simulink model "mfordmodel_v1"  (R2023a)
settings: Solver=ode45  StartTime=0.0  StopTime=10.0  RelTol=1e-3  EnableMultiTasking=on
undefined symbols (not defined in the file): ABV_RATIO_SW, AC_OFF_DLY, ACLOD, AUTO_TRNS_SW, BRAKE_DNDT_X, BZZRPM, BZZRPM_ALT, BZZTM, BZZTM_ALT, CMD_LITOFF, CMD_STABLE, CO_ST_ECT__A, COOL_BASE, DAS_BKDLY_A, DAS_CNT, DAS_CTDLY, DAS_LC_SW__A, DASCLP_5INH, DASCTL, DASMHYST, DASMPH, DEBYCP, DES_BASE, DPNEU_MUL, DSDRPM_DN_TC, DSDRPM_OFF, DSDRPM_UP_TC, EDF_DELAY, EDFHP, ETC_CL_TP, ETC_HP, GR_CM_CREEP, HCAM_ACT_CLP, HEDFHP, HEDFRPM, HICAM_PS, IAC_CAL_SW, IAC_ER_TM1, IAC_ER_TM2, IAC_ER_TM4, IAC_HI_LIM__A, IAC_ISFL_OBD, IAC_KAM_SW, IAC_LO_LIM__A, IAC_MON_TM, IAC_OT_REQ, IAC_RUN_TM, IAC_TP_OBD, IAC_TR_DAS, IAC_TST_DC, ID_DAS__A, ID_NOVS__A, IDVS_CH__A, IDVS_SL__A, IPSI_SW, IPSIDLY, IS_DRBASE__A, IS_DRBASE_A__A, IS_NUBASE__A, IS_NUBASE_A__A ... (+35)
libraries: simulink x2
(part 7 of 12)

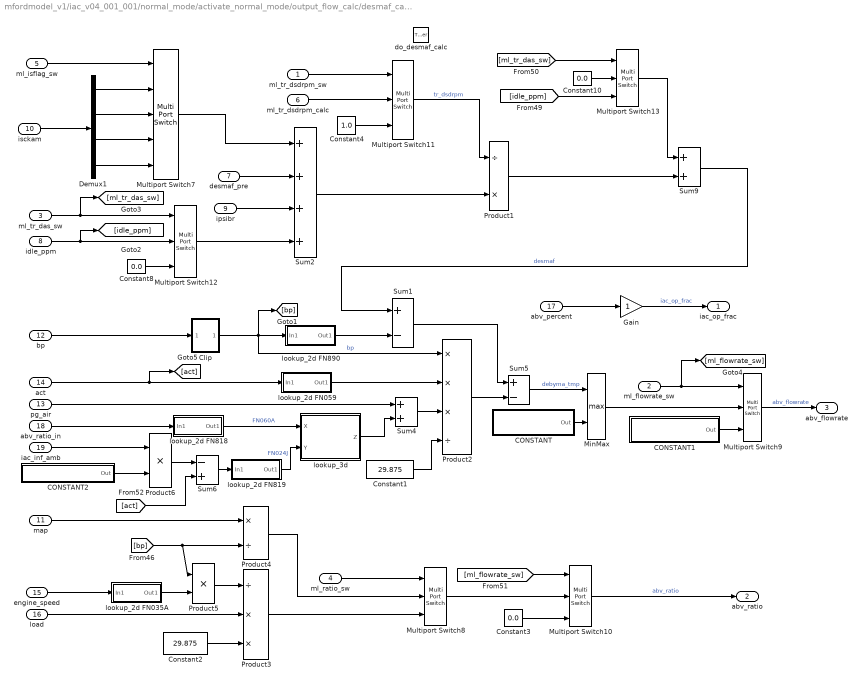
== system mfordmodel_v1/iac_v04_001_001/normal_mode/activate_normal_mode/output_flow_calc/desmaf_calc ==
  ml_tr_dsdrpm_sw : Inport
  ml_flowrate_sw : Inport  Port=2
  ml_tr_das_sw : Inport  Port=3
  ml_ratio_sw : Inport  Port=4
  ml_isflag_sw : Inport  Port=5
  ml_tr_dsdrpm_calc : Inport  Port=6
  desmaf_pre : Inport  Port=7
  idle_ppm : Inport  Port=8
  ipsibr : Inport  Port=9
  isckam : Inport  Port=10
  map : Inport  Port=11
  bp : Inport  Port=12
  pg_air : Inport  Port=13
  act : Inport  Port=14
  engine_speed : Inport  Port=15
  load : Inport  Port=16
  abv_percent : Inport  Port=17
  abv_ratio_in : Inport  Port=18
  iac_inf_amb : Inport  Port=19
  do_desmaf_calc : TriggerPort  TriggerType=function-call  VariantControl=(inherit)
  CONSTANT : Subsystem  mask(Constant){constant=DEBYCP}
      mask help: Constant Block. Will dispaly constant name and value on the icon of the block
      mask init:
      | if isletter(constant(1))
      |   const = evalin('base',constant);
      |   name = constant;
      | else
      |   const = str2num(constant);
      |   name = 'CONST';
      | end;
      mask Display: fprintf('%s = %.4f',name,const);
  CONSTANT1 : Subsystem  mask(Constant){constant=IAC_FM_PPM}
      mask help: Constant Block. Will dispaly constant name and value on the icon of the block
      mask init:
      | if isletter(constant(1))
      |   const = evalin('base',constant);
      |   name = constant;
      | else
      |   const = str2num(constant);
      |   name = 'CONST';
      | end;
      mask Display: fprintf('%s = %.4f',name,const);
  CONSTANT2 : Subsystem  mask(Constant){constant=LK_AMB_FRAC}
      mask help: Constant Block. Will dispaly constant name and value on the icon of the block
      mask init:
      | if isletter(constant(1))
      |   const = evalin('base',constant);
      |   name = constant;
      | else
      |   const = str2num(constant);
      |   name = 'CONST';
      | end;
      mask Display: fprintf('%s = %.4f',name,const);
  Clip : Subsystem  mask(Clip){max=40, min=.1, labels=on}
      mask prompts: max "Upper Limit"; min "Lower Limit"; labels "Show clip values"
      mask help:
      | Limits input signal to the upper and lower saturation
      | values.
      mask init:
      | if (labels == 1)
      |   up_label = num2str(max, '%5.3g');
      |   low_label = num2str(min, '%5.3g');
      | else
      |   up_label = ' ';
      |   low_label = ' ';
      | end
      mask Help:
      | Upper limit  -  The upper bound on the input signal.  While the signal is above this value, the block output is set to this value.
      | 
      | Lower limit  -  The lower bound on the input signal.  While the signal is below this value, the block output is set to this value.
      | 
      | Show clip values  -  If the box is checked, clip values are displayed in the icon box.
      mask Display:
      | plot( [0.1 0.3 0.7 0.9], [0.2 0.2 0.8 0.8])
      | text(0.2, 0.05, low_label)
      | text(0.7, 0.95, up_label)
  Constant1 : Constant  Value=29.875
  Constant10 : Constant  Value=0.0
  Constant2 : Constant  Value=29.875
  Constant3 : Constant  Value=0.0
  Constant4 : Constant  Value=1.0
  Constant8 : Constant  Value=0.0
  Demux1 : Demux
      settings: DisplayOption=none
  Gain : Gain  SaturateOnIntegerOverflow=on  OutDataTypeStr=Inherit: Same as input  ParamDataTypeStr=Inherit: Same as input
  MinMax : MinMax  Function=max  Inputs=2  InputSameDT=on  SaturateOnIntegerOverflow=on
  Multiport Switch{8..13} (6 alike) : MultiPortSwitch  Inputs=2
  Multiport Switch7 : MultiPortSwitch  Inputs=4
  Product1 : Product  Inputs=/*  InputSameDT=on  RndMeth=Zero  SaturateOnIntegerOverflow=on  OutDataTypeStr=Inherit: Same as first input
  Product2 : Product  Inputs=***/  InputSameDT=on  RndMeth=Zero  SaturateOnIntegerOverflow=on  OutDataTypeStr=Inherit: Same as first input
  Product3 : Product  Inputs=/**  InputSameDT=on  RndMeth=Zero  SaturateOnIntegerOverflow=on  OutDataTypeStr=Inherit: Same as first input
  Product4 : Product  Inputs=*/  InputSameDT=on  RndMeth=Zero  SaturateOnIntegerOverflow=on  OutDataTypeStr=Inherit: Same as first input
  Product5 : Product  Inputs=**  InputSameDT=on  RndMeth=Zero  SaturateOnIntegerOverflow=on  OutDataTypeStr=Inherit: Same as first input
  Product6 : Product  Inputs=**  InputSameDT=on  RndMeth=Zero  SaturateOnIntegerOverflow=on  OutDataTypeStr=Inherit: Same as first input
  Sum1 : Sum  Inputs=+-  InputSameDT=on  SaturateOnIntegerOverflow=on  OutDataTypeStr=Inherit: Same as first input
  Sum2 : Sum  Inputs=++++  InputSameDT=on  SaturateOnIntegerOverflow=on  OutDataTypeStr=Inherit: Same as first input
  Sum4 : Sum  InputSameDT=on  SaturateOnIntegerOverflow=on  OutDataTypeStr=Inherit: Same as first input
  Sum5 : Sum  Inputs=+-  InputSameDT=on  SaturateOnIntegerOverflow=on  OutDataTypeStr=Inherit: Same as first input
  Sum6 : Sum  Inputs=-+  InputSameDT=on  SaturateOnIntegerOverflow=on  OutDataTypeStr=Inherit: Same as first input
  Sum9 : Sum  InputSameDT=on  SaturateOnIntegerOverflow=on  OutDataTypeStr=Inherit: Same as first input
  lookup_2d FN035A : Subsystem  mask(2-D, piece-wise, linear interpolation){CAL_FUNC=FN035A}
      mask prompts: CAL_FUNC "Calibration function name"
      mask help:
      | Performs piece-wise linear interpolation.
      |
      | Output is NOT extrapolated beyond the input range.  If the input value presented to the block lies outside the range specified in the block's parameter, then the value is treated as though it has the value of the nearest value in the range.
      mask init: same as mfordmodel_v1/iac_v04_001_001/activate_desired_rpm/rpm_calcs/lookup_2d
      mask Help:
      | Enter the name of the calibration function.
      | (e.g. EGM_VA_ECT_MULT)
      mask Display:
      | fprintf('%s',CAL_FUNC);
      | plot(calfunc.X,calfunc.Y,max_x*1.05,max_y*1.05,min_x,min_y);
  lookup_2d FN059 : Subsystem  mask(2-D, piece-wise, linear interpolation){CAL_FUNC=FN059}
      mask prompts: CAL_FUNC "Calibration function name"
      mask help:
      | Performs piece-wise linear interpolation.
      |
      | Output is NOT extrapolated beyond the input range.  If the input value presented to the block lies outside the range specified in the block's parameter, then the value is treated as though it has the value of the nearest value in the range.
      mask init: same as mfordmodel_v1/iac_v04_001_001/activate_desired_rpm/rpm_calcs/lookup_2d
      mask Help:
      | Enter the name of the calibration function.
      | (e.g. EGM_VA_ECT_MULT)
      mask Display:
      | fprintf('%s',CAL_FUNC);
      | plot(calfunc.X,calfunc.Y,max_x*1.05,max_y*1.05,min_x,min_y);
  lookup_2d FN818 : Subsystem  mask(2-D, piece-wise, linear interpolation){CAL_FUNC=FN060A}
      mask prompts: CAL_FUNC "Calibration function name"
      mask help:
      | Performs piece-wise linear interpolation.
      |
      | Output is NOT extrapolated beyond the input range.  If the input value presented to the block lies outside the range specified in the block's parameter, then the value is treated as though it has the value of the nearest value in the range.
      mask init: same as mfordmodel_v1/iac_v04_001_001/activate_desired_rpm/rpm_calcs/lookup_2d
      mask Help:
      | Enter the name of the calibration function.
      | (e.g. EGM_VA_ECT_MULT)
      mask Display:
      | fprintf('%s',CAL_FUNC);
      | plot(calfunc.X,calfunc.Y,max_x*1.05,max_y*1.05,min_x,min_y);
  lookup_2d FN819 : Subsystem  mask(2-D, piece-wise, linear interpolation){CAL_FUNC=FN024J}
      mask prompts: CAL_FUNC "Calibration function name"
      mask help:
      | Performs piece-wise linear interpolation.
      |
      | Output is NOT extrapolated beyond the input range.  If the input value presented to the block lies outside the range specified in the block's parameter, then the value is treated as though it has the value of the nearest value in the range.
      mask init: same as mfordmodel_v1/iac_v04_001_001/activate_desired_rpm/rpm_calcs/lookup_2d
      mask Help:
      | Enter the name of the calibration function.
      | (e.g. EGM_VA_ECT_MULT)
      mask Display:
      | fprintf('%s',CAL_FUNC);
      | plot(calfunc.X,calfunc.Y,max_x*1.05,max_y*1.05,min_x,min_y);
  lookup_2d FN890 : Subsystem  mask(2-D, piece-wise, linear interpolation){CAL_FUNC=FN890}
      mask prompts: CAL_FUNC "Calibration function name"
      mask help:
      | Performs piece-wise linear interpolation.
      |
      | Output is NOT extrapolated beyond the input range.  If the input value presented to the block lies outside the range specified in the block's parameter, then the value is treated as though it has the value of the nearest value in the range.
      mask init: same as mfordmodel_v1/iac_v04_001_001/activate_desired_rpm/rpm_calcs/lookup_2d
      mask Help:
      | Enter the name of the calibration function.
      | (e.g. EGM_VA_ECT_MULT)
      mask Display:
      | fprintf('%s',CAL_FUNC);
      | plot(calfunc.X,calfunc.Y,max_x*1.05,max_y*1.05,min_x,min_y);
  lookup_3d : Subsystem  mask(3-D, piece-wise, linear interpolation){CAL_TABLE=FN8180}
      mask prompts: CAL_TABLE "Calibration table name"
      mask help:
      | Performs 3-D, piece-wise linear interpolation.
      |
      | Output is NOT extrapolated beyond the input ranges.  If an input value presented to the block lies outside the range specified in the block's parameters, then the value is treated as though it has the value of the nearest value in the range.
      mask init: same as mfordmodel_v1/iac_v04_001_001/normal_mode/activate_feedforward/desmaf_pre_calc/FN1862AD
      mask Help: Enter the name of the calibration table.
      mask Display:
      | fprintf('%s',CAL_TABLE);
      | plot(caltable.Z');
      | plot([min_x max_x],[minz*.99 minz*.99]);
      | plot([min_x min_x],[minz*.99 maxz*1.01]);
  iac_op_frac : Outport
  abv_ratio : Outport  Port=2
  abv_flowrate : Outport  Port=3
  wires:
  Multiport Switch7/1 -> Sum2/1
  Demux1/1 -> Multiport Switch7/2
  Demux1/2 -> Multiport Switch7/3
  Demux1/3 -> Multiport Switch7/4
  Demux1/4 -> Multiport Switch7/5
  ml_isflag_sw/1 -> Multiport Switch7/1
  isckam/1 -> Demux1/1
  Constant8/1 -> Multiport Switch12/3
  desmaf_pre/1 -> Sum2/2
  Multiport Switch11/1 -> Product1/1  "tr_dsdrpm"
  Sum2/1 -> Product1/2
  ipsibr/1 -> Sum2/3
  Multiport Switch13/1 -> Sum9/1
  Product1/1 -> Sum9/2
  Multiport Switch12/1 -> Sum2/4
  Constant10/1 -> Multiport Switch13/2
  [idle_ppm] -> Multiport Switch13/3
  Constant4/1 -> Multiport Switch11/3
  ml_tr_dsdrpm_sw/1 -> Multiport Switch11/1
  ml_tr_dsdrpm_calc/1 -> Multiport Switch11/2
  [ml_tr_das_sw] -> Multiport Switch13/1
  ml_tr_das_sw/1 -> Multiport Switch12/1, [ml_tr_das_sw]
  idle_ppm/1 -> [idle_ppm], Multiport Switch12/2
  ml_ratio_sw/1 -> Multiport Switch8/1
  Product4/1 -> Multiport Switch8/2
  Product3/1 -> Multiport Switch8/3
  Multiport Switch8/1 -> Multiport Switch10/2
  [ml_flowrate_sw] -> Multiport Switch10/1
  Constant3/1 -> Multiport Switch10/3
  map/1 -> Product4/1
  Product5/1 -> Product3/1
  [bp] -> Product4/2, Product5/1
  load/1 -> Product3/2
  engine_speed/1 -> lookup_2d FN035A/1(In1)
  Constant2/1 -> Product3/3
  lookup_2d FN035A/1(Out1) -> Product5/2
  Multiport Switch10/1 -> abv_ratio/1  "abv_ratio"
  MinMax/1 -> Multiport Switch9/2
  CONSTANT1/1(Out) -> Multiport Switch9/3
  Multiport Switch9/1 -> abv_flowrate/1  "abv_flowrate"
  Sum5/1 -> MinMax/1  "debyma_tmp"
  CONSTANT/1(Out) -> MinMax/2
  Product2/1 -> Sum5/2
  Sum1/1 -> Sum5/1
  lookup_2d FN890/1(Out1) -> Sum1/2
  Constant1/1 -> Product2/4
  Sum9/1 -> Sum1/1  "desmaf"
  ml_flowrate_sw/1 -> Multiport Switch9/1, [ml_flowrate_sw]
  Sum4/1 -> Product2/3
  pg_air/1 -> Sum4/1
  lookup_2d FN059/1(Out1) -> Product2/2
  bp/1 -> Clip/1(In1)
  Clip/1(Out1) -> [bp], Product2/1, lookup_2d FN890/1(In1)  "bp"
  abv_ratio_in/1 -> lookup_2d FN818/1(In1)
  lookup_3d/1(Z) -> Sum4/2
  lookup_2d FN818/1(Out1) -> lookup_3d/1(X)  "FN060A"
  act/1 -> lookup_2d FN059/1(In1), [act]
  iac_inf_amb/1 -> Product6/1
  Product6/1 -> Sum6/1
  [act] -> Sum6/2
  Sum6/1 -> lookup_2d FN819/1(In1)
  lookup_2d FN819/1(Out1) -> lookup_3d/2(Y)  "FN024J"
  Gain/1 -> iac_op_frac/1  "iac_op_frac"
  abv_percent/1 -> Gain/1
  CONSTANT2/1(Out) -> Product6/2

== system mfordmodel_v1/iac_v04_001_001/normal_mode/activate_normal_mode/output_flow_calc/tr_dsdrpm_calc ==
  tr_abs : Inport
  tr_res : Inport  Port=2
  do_tr_dsdrpm_calc : TriggerPort  TriggerType=function-call  VariantControl=(inherit)
  Sum1 : Sum  Inputs=+-  InputSameDT=on  SaturateOnIntegerOverflow=on  OutDataTypeStr=Inherit: Same as first input
  ml_tr_dsdrpm_calc : Outport  InitialOutput=0
  wires:
  tr_abs/1 -> Sum1/1
  Sum1/1 -> ml_tr_dsdrpm_calc/1  "ml_tr_dsdrpm_calc"
  tr_res/1 -> Sum1/2

== system mfordmodel_v1/iac_v04_001_001/normal_mode/iscflg_module/das_min_clip/functions ==
  n_ratch : Inport
  dasl_min_clp : Inport  Port=2
  iac_dlt_time : Inport  Port=3
  dsdrpm : Inport  Port=4
  do_functions : TriggerPort  TriggerType=function-call  VariantControl=(inherit)
  ROLAV_TC_DT_in1 : Subsystem  mask(Rolling Average - Time Constant){TAU=TC_DAS_CLPUC}
      mask prompts: TAU "Time Constant"
      mask help: Rolling Average - Time Constant. This filter block is the first order approximation using a time constant. Inputs include the time constant (entered through this dialogue), old_ave which is the previous average value, new_value which is the new filter to filter toward, and the delta_time which is elapsed time over which to perform the filter equation.
      mask init:
      | if isletter(TAU(1))
      |   tc = evalin('base',TAU);
      |   name = TAU;
      | else
      |   tc = str2num(TAU);
      |   name = 'TC';
      | end;
      mask Display: fprintf('%s = %.4f',name,tc);
  ROLAV_TC_DT_in2 : Subsystem  mask(Rolling Average - Time Constant){TAU=TC_DAS_CLPLC}
      mask prompts: TAU "Time Constant"
      mask help: Rolling Average - Time Constant. This filter block is the first order approximation using a time constant. Inputs include the time constant (entered through this dialogue), old_ave which is the previous average value, new_value which is the new filter to filter toward, and the delta_time which is elapsed time over which to perform the filter equation.
      mask init:
      | if isletter(TAU(1))
      |   tc = evalin('base',TAU);
      |   name = TAU;
      | else
      |   tc = str2num(TAU);
      |   name = 'TC';
      | end;
      mask Display: fprintf('%s = %.4f',name,tc);
  ROLAV_TC_DT_in3 : Subsystem  mask(Rolling Average - Time Constant){TAU=TC_DAS_CLPUC}
      mask prompts: TAU "Time Constant"
      mask help: Rolling Average - Time Constant. This filter block is the first order approximation using a time constant. Inputs include the time constant (entered through this dialogue), old_ave which is the previous average value, new_value which is the new filter to filter toward, and the delta_time which is elapsed time over which to perform the filter equation.
      mask init:
      | if isletter(TAU(1))
      |   tc = evalin('base',TAU);
      |   name = TAU;
      | else
      |   tc = str2num(TAU);
      |   name = 'TC';
      | end;
      mask Display: fprintf('%s = %.4f',name,tc);
  ROLAV_TC_DT_in4 : Subsystem  mask(Rolling Average - Time Constant){TAU=TC_DAS_CLPLC}
      mask prompts: TAU "Time Constant"
      mask help: Rolling Average - Time Constant. This filter block is the first order approximation using a time constant. Inputs include the time constant (entered through this dialogue), old_ave which is the previous average value, new_value which is the new filter to filter toward, and the delta_time which is elapsed time over which to perform the filter equation.
      mask init:
      | if isletter(TAU(1))
      |   tc = evalin('base',TAU);
      |   name = TAU;
      | else
      |   tc = str2num(TAU);
      |   name = 'TC';
      | end;
      mask Display: fprintf('%s = %.4f',name,tc);
  Sum2 : Sum  Inputs=-+  InputSameDT=on  SaturateOnIntegerOverflow=on  OutDataTypeStr=Inherit: Same as first input
  lookup_2d3 : Subsystem  mask(2-D, piece-wise, linear interpolation){CAL_FUNC=FN894}
      mask prompts: CAL_FUNC "Calibration function name"
      mask help:
      | Performs piece-wise linear interpolation.
      |
      | Output is NOT extrapolated beyond the input range.  If the input value presented to the block lies outside the range specified in the block's parameter, then the value is treated as though it has the value of the nearest value in the range.
      mask init: same as mfordmodel_v1/iac_v04_001_001/activate_desired_rpm/rpm_calcs/lookup_2d
      mask Help:
      | Enter the name of the calibration function.
      | (e.g. EGM_VA_ECT_MULT)
      mask Display:
      | fprintf('%s',CAL_FUNC);
      | plot(calfunc.X,calfunc.Y,max_x*1.05,max_y*1.05,min_x,min_y);
  lookup_2d6 : Subsystem  mask(2-D, piece-wise, linear interpolation){CAL_FUNC=FN894LLC}
      mask prompts: CAL_FUNC "Calibration function name"
      mask help:
      | Performs piece-wise linear interpolation.
      |
      | Output is NOT extrapolated beyond the input range.  If the input value presented to the block lies outside the range specified in the block's parameter, then the value is treated as though it has the value of the nearest value in the range.
      mask init: same as mfordmodel_v1/iac_v04_001_001/activate_desired_rpm/rpm_calcs/lookup_2d
      mask Help:
      | Enter the name of the calibration function.
      | (e.g. EGM_VA_ECT_MULT)
      mask Display:
      | fprintf('%s',CAL_FUNC);
      | plot(calfunc.X,calfunc.Y,max_x*1.05,max_y*1.05,min_x,min_y);
  lookup_2d7 : Subsystem  mask(2-D, piece-wise, linear interpolation){CAL_FUNC=FN894HLC}
      mask prompts: CAL_FUNC "Calibration function name"
      mask help:
      | Performs piece-wise linear interpolation.
      |
      | Output is NOT extrapolated beyond the input range.  If the input value presented to the block lies outside the range specified in the block's parameter, then the value is treated as though it has the value of the nearest value in the range.
      mask init: same as mfordmodel_v1/iac_v04_001_001/activate_desired_rpm/rpm_calcs/lookup_2d
      mask Help:
      | Enter the name of the calibration function.
      | (e.g. EGM_VA_ECT_MULT)
      mask Display:
      | fprintf('%s',CAL_FUNC);
      | plot(calfunc.X,calfunc.Y,max_x*1.05,max_y*1.05,min_x,min_y);
  lookup_2d8 : Subsystem  mask(2-D, piece-wise, linear interpolation){CAL_FUNC=FN894L}
      mask prompts: CAL_FUNC "Calibration function name"
      mask help:
      | Performs piece-wise linear interpolation.
      |
      | Output is NOT extrapolated beyond the input range.  If the input value presented to the block lies outside the range specified in the block's parameter, then the value is treated as though it has the value of the nearest value in the range.
      mask init: same as mfordmodel_v1/iac_v04_001_001/activate_desired_rpm/rpm_calcs/lookup_2d
      mask Help:
      | Enter the name of the calibration function.
      | (e.g. EGM_VA_ECT_MULT)
      mask Display:
      | fprintf('%s',CAL_FUNC);
      | plot(calfunc.X,calfunc.Y,max_x*1.05,max_y*1.05,min_x,min_y);
  lookup_2d9 : Subsystem  mask(2-D, piece-wise, linear interpolation){CAL_FUNC=FN894H}
      mask prompts: CAL_FUNC "Calibration function name"
      mask help:
      | Performs piece-wise linear interpolation.
      |
      | Output is NOT extrapolated beyond the input range.  If the input value presented to the block lies outside the range specified in the block's parameter, then the value is treated as though it has the value of the nearest value in the range.
      mask init: same as mfordmodel_v1/iac_v04_001_001/activate_desired_rpm/rpm_calcs/lookup_2d
      mask Help:
      | Enter the name of the calibration function.
      | (e.g. EGM_VA_ECT_MULT)
      mask Display:
      | fprintf('%s',CAL_FUNC);
      | plot(calfunc.X,calfunc.Y,max_x*1.05,max_y*1.05,min_x,min_y);
  ml_rolav_hlc : Outport
  ml_rolav_llc : Outport  Port=2
  ml_rolav_l : Outport  Port=3
  ml_rolav_h : Outport  Port=4
  ml_fn894 : Outport  Port=5
  ml_fn894l : Outport  Port=6
  ml_fn894h : Outport  Port=7
  ml_fn894llc : Outport  Port=8
  ml_fn894hlc : Outport  Port=9
  wires:
  ROLAV_TC_DT_in3/1(new_ave) -> ml_rolav_h/1  "ml_rolav_h"
  [fn894h] -> ROLAV_TC_DT_in3/1(new_value)
  lookup_2d7/1(Out1) -> [fn894hlc], ml_fn894hlc/1  "ml_fn894hlc"
  lookup_2d9/1(Out1) -> [fn894h], ml_fn894h/1  "ml_fn894h"
  ROLAV_TC_DT_in2/1(new_ave) -> ml_rolav_hlc/1  "ml_rolav_hlc"
  [fn894hlc] -> ROLAV_TC_DT_in2/1(new_value)
  iac_dlt_time/1 -> ROLAV_TC_DT_in3/3(delta_time), ROLAV_TC_DT_in2/3(delta_time), ROLAV_TC_DT_in1/3(delta_time), ROLAV_TC_DT_in4/3(delta_time)
  dasl_min_clp/1 -> ROLAV_TC_DT_in3/2(old_ave), ROLAV_TC_DT_in2/2(old_ave), ROLAV_TC_DT_in1/2(old_ave), ROLAV_TC_DT_in4/2(old_ave)
  [fn894l] -> ROLAV_TC_DT_in1/1(new_value)
  ROLAV_TC_DT_in1/1(new_ave) -> ml_rolav_l/1  "ml_rolav_l"
  ROLAV_TC_DT_in4/1(new_ave) -> ml_rolav_llc/1  "ml_rolav_llc"
  [fn894llc] -> ROLAV_TC_DT_in4/1(new_value)
  lookup_2d8/1(Out1) -> [fn894l], ml_fn894l/1  "ml_fn894l"
  lookup_2d6/1(Out1) -> [fn894llc], ml_fn894llc/1  "ml_fn894llc"
  Sum2/1 -> lookup_2d8/1(In1), lookup_2d9/1(In1), lookup_2d6/1(In1), lookup_2d7/1(In1), lookup_2d3/1(In1)
  lookup_2d3/1(Out1) -> ml_fn894/1  "ml_fn894"
  dsdrpm/1 -> Sum2/1
  n_ratch/1 -> Sum2/2

== system mfordmodel_v1/iac_v04_001_001/normal_mode/iscflg_module/dashpot/TIMER ==
  note: Timer Control calls functions within the Time Calculator
      | after using the flags 'increment_flag' and 'decrement_flag'
      | to determine the direction of the timer.
  note: timer14/TIMER
  trig_time : Inport
  trig_reset : Inport  Port=2
  reset value : Inport  Port=3
  inc flag : Inport  Port=4
  dec flag : Inport  Port=5
  Event Triggers : Mux  Inputs=2
  Time Calculator : Subsystem
  Timer Control : Stateflow chart  TreatAsAtomicUnit=on
  timer : Outport
  wires:
  reset value/1 -> Time Calculator/5(reset_value)  "reset_value"
  trig_reset/1 -> Event Triggers/2  "trig_reset"
  trig_time/1 -> Event Triggers/1  "trig_timer"
  Event Triggers/1 -> Timer Control/Trigger
  Time Calculator/1(timer) -> timer/1  "timer"
  Timer Control/1(count_direction) -> Time Calculator/1(count_direction)  "count_direction"
  Timer Control/2(reset_flag) -> Time Calculator/2(reset_val)  "reset_flag"
  Timer Control/3(do_delta_time()) -> Time Calculator/3(do_delta_time)  "do_delta_time"
  Timer Control/4(do_timer()) -> Time Calculator/4(do_timer)  "do_timer"
  dec flag/1 -> Timer Control/2(decr_flag)  "decrement_flag"
  inc flag/1 -> Timer Control/1(incr_flag)  "increment_flag"

== system mfordmodel_v1/iac_v04_001_001/normal_mode/iscflg_module/dashpot/daspot_calc ==
  ml_idle_ppm_sw : Inport
  iac_dlt_time : Inport  Port=2
  idle_ppm_in : Inport  Port=3
  das_ppm__A : Inport  Port=4
  das_tc__A : Inport  Port=5
  do_daspot_calc : TriggerPort  TriggerType=function-call  VariantControl=(inherit)
  Constant : Constant  Value=0
  Constant1 : Constant  Value=0
  MinMax : MinMax  Function=max  Inputs=2  InputSameDT=on  SaturateOnIntegerOverflow=on
  MinMax1 : MinMax  Function=max  Inputs=2  InputSameDT=on  SaturateOnIntegerOverflow=on
  Multiport Switch : MultiPortSwitch
  ROLAV_TC_in_DT_in : Subsystem  mask(Rolling Average - Time Constant){}
      mask help: Rolling Average - Time Constant. This filter block is the first order approximation using a time constant. Inputs include the time constant, old_ave which is the previous average value, new_value which is the new filter to filter toward, and the delta_time which is elapsed time over which to perform the filter equation.
      mask Display: fprintf('ROLAV_TC');
  Sum : Sum  Inputs=-+  InputSameDT=on  SaturateOnIntegerOverflow=on  OutDataTypeStr=Inherit: Same as first input
  Sum1 : Sum  Inputs=-+  InputSameDT=on  SaturateOnIntegerOverflow=on  OutDataTypeStr=Inherit: Same as first input
  lookup_2d : Subsystem  mask(2-D, piece-wise, linear interpolation){CAL_FUNC=FN879}
      mask prompts: CAL_FUNC "Calibration function name"
      mask help:
      | Performs piece-wise linear interpolation.
      |
      | Output is NOT extrapolated beyond the input range.  If the input value presented to the block lies outside the range specified in the block's parameter, then the value is treated as though it has the value of the nearest value in the range.
      mask init: same as mfordmodel_v1/iac_v04_001_001/activate_desired_rpm/rpm_calcs/lookup_2d
      mask Help:
      | Enter the name of the calibration function.
      | (e.g. EGM_VA_ECT_MULT)
      mask Display:
      | fprintf('%s',CAL_FUNC);
      | plot(calfunc.X,calfunc.Y,max_x*1.05,max_y*1.05,min_x,min_y);
  lookup_2d2 : Subsystem  mask(2-D, piece-wise, linear interpolation){CAL_FUNC=FN879LC}
      mask prompts: CAL_FUNC "Calibration function name"
      mask help:
      | Performs piece-wise linear interpolation.
      |
      | Output is NOT extrapolated beyond the input range.  If the input value presented to the block lies outside the range specified in the block's parameter, then the value is treated as though it has the value of the nearest value in the range.
      mask init: same as mfordmodel_v1/iac_v04_001_001/activate_desired_rpm/rpm_calcs/lookup_2d
      mask Help:
      | Enter the name of the calibration function.
      | (e.g. EGM_VA_ECT_MULT)
      mask Display:
      | fprintf('%s',CAL_FUNC);
      | plot(calfunc.X,calfunc.Y,max_x*1.05,max_y*1.05,min_x,min_y);
  idle_ppm : Outport
  wires:
  Multiport Switch/1 -> idle_ppm/1  "idle_ppm"
  MinMax/1 -> Multiport Switch/3
  Constant1/1 -> MinMax/2
  Sum1/1 -> MinMax/1
  MinMax1/1 -> Multiport Switch/4
  Constant/1 -> MinMax1/2
  Sum/1 -> MinMax1/1
  lookup_2d2/1(Out1) -> Sum1/1
  lookup_2d/1(Out1) -> Sum/1
  iac_dlt_time/1 -> ROLAV_TC_in_DT_in/4(delta_time)
  ROLAV_TC_in_DT_in/1(new_ave) -> Multiport Switch/2
  das_tc__A/1 -> ROLAV_TC_in_DT_in/2(Tau)
  idle_ppm_in/1 -> Sum1/2, Sum/2, lookup_2d/1(In1), lookup_2d2/1(In1), ROLAV_TC_in_DT_in/3(old_ave)
  das_ppm__A/1 -> ROLAV_TC_in_DT_in/1(new_value)
  ml_idle_ppm_sw/1 -> Multiport Switch/1

== system mfordmodel_v1/iac_v04_001_001/normal_mode/iscflg_module/dashpot/function_calcs ==
  engine_speed : Inport
  vsbart : Inport  Port=2
  do_function_calcs : TriggerPort  TriggerType=function-call  VariantControl=(inherit)
  lookup_2d : Subsystem  mask(2-D, piece-wise, linear interpolation){CAL_FUNC=FNBO12}
      mask prompts: CAL_FUNC "Calibration function name"
      mask help:
      | Performs piece-wise linear interpolation.
      |
      | Output is NOT extrapolated beyond the input range.  If the input value presented to the block lies outside the range specified in the block's parameter, then the value is treated as though it has the value of the nearest value in the range.
      mask init: same as mfordmodel_v1/iac_v04_001_001/activate_desired_rpm/rpm_calcs/lookup_2d
      mask Help:
      | Enter the name of the calibration function.
      | (e.g. EGM_VA_ECT_MULT)
      mask Display:
      | fprintf('%s',CAL_FUNC);
      | plot(calfunc.X,calfunc.Y,max_x*1.05,max_y*1.05,min_x,min_y);
  lookup_2d1 : Subsystem  mask(2-D, piece-wise, linear interpolation){CAL_FUNC=FNBO13}
      mask prompts: CAL_FUNC "Calibration function name"
      mask help:
      | Performs piece-wise linear interpolation.
      |
      | Output is NOT extrapolated beyond the input range.  If the input value presented to the block lies outside the range specified in the block's parameter, then the value is treated as though it has the value of the nearest value in the range.
      mask init: same as mfordmodel_v1/iac_v04_001_001/activate_desired_rpm/rpm_calcs/lookup_2d
      mask Help:
      | Enter the name of the calibration function.
      | (e.g. EGM_VA_ECT_MULT)
      mask Display:
      | fprintf('%s',CAL_FUNC);
      | plot(calfunc.X,calfunc.Y,max_x*1.05,max_y*1.05,min_x,min_y);
  lookup_2d2 : Subsystem  mask(2-D, piece-wise, linear interpolation){CAL_FUNC=FNBO23}
      mask prompts: CAL_FUNC "Calibration function name"
      mask help:
      | Performs piece-wise linear interpolation.
      |
      | Output is NOT extrapolated beyond the input range.  If the input value presented to the block lies outside the range specified in the block's parameter, then the value is treated as though it has the value of the nearest value in the range.
      mask init: same as mfordmodel_v1/iac_v04_001_001/activate_desired_rpm/rpm_calcs/lookup_2d
      mask Help:
      | Enter the name of the calibration function.
      | (e.g. EGM_VA_ECT_MULT)
      mask Display:
      | fprintf('%s',CAL_FUNC);
      | plot(calfunc.X,calfunc.Y,max_x*1.05,max_y*1.05,min_x,min_y);
  lookup_2d3 : Subsystem  mask(2-D, piece-wise, linear interpolation){CAL_FUNC=FN899}
      mask prompts: CAL_FUNC "Calibration function name"
      mask help:
      | Performs piece-wise linear interpolation.
      |
      | Output is NOT extrapolated beyond the input range.  If the input value presented to the block lies outside the range specified in the block's parameter, then the value is treated as though it has the value of the nearest value in the range.
      mask init: same as mfordmodel_v1/iac_v04_001_001/activate_desired_rpm/rpm_calcs/lookup_2d
      mask Help:
      | Enter the name of the calibration function.
      | (e.g. EGM_VA_ECT_MULT)
      mask Display:
      | fprintf('%s',CAL_FUNC);
      | plot(calfunc.X,calfunc.Y,max_x*1.05,max_y*1.05,min_x,min_y);
  lookup_2d4 : Subsystem  mask(2-D, piece-wise, linear interpolation){CAL_FUNC=FNBO24}
      mask prompts: CAL_FUNC "Calibration function name"
      mask help:
      | Performs piece-wise linear interpolation.
      |
      | Output is NOT extrapolated beyond the input range.  If the input value presented to the block lies outside the range specified in the block's parameter, then the value is treated as though it has the value of the nearest value in the range.
      mask init: same as mfordmodel_v1/iac_v04_001_001/activate_desired_rpm/rpm_calcs/lookup_2d
      mask Help:
      | Enter the name of the calibration function.
      | (e.g. EGM_VA_ECT_MULT)
      mask Display:
      | fprintf('%s',CAL_FUNC);
      | plot(calfunc.X,calfunc.Y,max_x*1.05,max_y*1.05,min_x,min_y);
  lookup_2d5 : Subsystem  mask(2-D, piece-wise, linear interpolation){CAL_FUNC=FNBO34}
      mask prompts: CAL_FUNC "Calibration function name"
      mask help:
      | Performs piece-wise linear interpolation.
      |
      | Output is NOT extrapolated beyond the input range.  If the input value presented to the block lies outside the range specified in the block's parameter, then the value is treated as though it has the value of the nearest value in the range.
      mask init: same as mfordmodel_v1/iac_v04_001_001/activate_desired_rpm/rpm_calcs/lookup_2d
      mask Help:
      | Enter the name of the calibration function.
      | (e.g. EGM_VA_ECT_MULT)
      mask Display:
      | fprintf('%s',CAL_FUNC);
      | plot(calfunc.X,calfunc.Y,max_x*1.05,max_y*1.05,min_x,min_y);
  lookup_2d6 : Subsystem  mask(2-D, piece-wise, linear interpolation){CAL_FUNC=FNBO35}
      mask prompts: CAL_FUNC "Calibration function name"
      mask help:
      | Performs piece-wise linear interpolation.
      |
      | Output is NOT extrapolated beyond the input range.  If the input value presented to the block lies outside the range specified in the block's parameter, then the value is treated as though it has the value of the nearest value in the range.
      mask init: same as mfordmodel_v1/iac_v04_001_001/activate_desired_rpm/rpm_calcs/lookup_2d
      mask Help:
      | Enter the name of the calibration function.
      | (e.g. EGM_VA_ECT_MULT)
      mask Display:
      | fprintf('%s',CAL_FUNC);
      | plot(calfunc.X,calfunc.Y,max_x*1.05,max_y*1.05,min_x,min_y);
  lookup_2d7 : Subsystem  mask(2-D, piece-wise, linear interpolation){CAL_FUNC=FNBO45}
      mask prompts: CAL_FUNC "Calibration function name"
      mask help:
      | Performs piece-wise linear interpolation.
      |
      | Output is NOT extrapolated beyond the input range.  If the input value presented to the block lies outside the range specified in the block's parameter, then the value is treated as though it has the value of the nearest value in the range.
      mask init: same as mfordmodel_v1/iac_v04_001_001/activate_desired_rpm/rpm_calcs/lookup_2d
      mask Help:
      | Enter the name of the calibration function.
      | (e.g. EGM_VA_ECT_MULT)
      mask Display:
      | fprintf('%s',CAL_FUNC);
      | plot(calfunc.X,calfunc.Y,max_x*1.05,max_y*1.05,min_x,min_y);
  ml_fnbo45 : Outport
  ml_fnbo35 : Outport  Port=2
  ml_fnbo34 : Outport  Port=3
  ml_fnbo24 : Outport  Port=4
  ml_fnbo23 : Outport  Port=5
  ml_fnbo13 : Outport  Port=6
  ml_fnbo12 : Outport  Port=7
  ml_fn899 : Outport  Port=8
  wires:
  vsbart/1 -> lookup_2d3/1(In1)
  lookup_2d3/1(Out1) -> ml_fn899/1  "ml_fn899"
  engine_speed/1 -> lookup_2d/1(In1), lookup_2d1/1(In1), lookup_2d2/1(In1), lookup_2d4/1(In1), lookup_2d5/1(In1), lookup_2d6/1(In1), lookup_2d7/1(In1)
  lookup_2d/1(Out1) -> ml_fnbo12/1  "ml_fnbo12"
  lookup_2d1/1(Out1) -> ml_fnbo13/1  "ml_fnbo13"
  lookup_2d2/1(Out1) -> ml_fnbo23/1  "ml_fnbo23"
  lookup_2d4/1(Out1) -> ml_fnbo24/1  "ml_fnbo24"
  lookup_2d5/1(Out1) -> ml_fnbo34/1  "ml_fnbo34"
  lookup_2d6/1(Out1) -> ml_fnbo35/1  "ml_fnbo35"
  lookup_2d7/1(Out1) -> ml_fnbo45/1  "ml_fnbo45"

== system mfordmodel_v1/iac_v04_001_001/normal_mode/iscflg_module/idle_drive_rpm_controller/idle_ppm_calc ==
  ml_idnerr : Inport
  idnerr_fil : Inport  Port=2
  ml_init_sw : Inport  Port=3
  ml_idnerr_sw : Inport  Port=4
  load : Inport  Port=5
  do_idle_ppm_calc : TriggerPort  TriggerType=function-call  VariantControl=(inherit)
  " 1" : Subsystem  mask(2-D, piece-wise, linear interpolation){CAL_FUNC=FN854}
      mask prompts: CAL_FUNC "Calibration function name"
      mask help:
      | Performs piece-wise linear interpolation.
      |
      | Output is NOT extrapolated beyond the input range.  If the input value presented to the block lies outside the range specified in the block's parameter, then the value is treated as though it has the value of the nearest value in the range.
      mask init: same as mfordmodel_v1/iac_v04_001_001/activate_desired_rpm/rpm_calcs/lookup_2d
      mask Help:
      | Enter the name of the calibration function.
      | (e.g. EGM_VA_ECT_MULT)
      mask Display:
      | fprintf('%s',CAL_FUNC);
      | plot(calfunc.X,calfunc.Y,max_x*1.05,max_y*1.05,min_x,min_y);
  CONSTANT7 : Subsystem  mask(Constant){constant=IDPROP_MIN__A}
      mask help: Constant Block. Will dispaly constant name and value on the icon of the block
      mask init:
      | if isletter(constant(1))
      |   const = evalin('base',constant);
      |   name = constant;
      | else
      |   const = str2num(constant);
      |   name = 'CONST';
      | end;
      mask Display: fprintf('%s = %.4f',name,const);
  CONSTANT8 : Subsystem  mask(Constant){constant=IDPROP_MAX__A}
      mask help: Constant Block. Will dispaly constant name and value on the icon of the block
      mask init:
      | if isletter(constant(1))
      |   const = evalin('base',constant);
      |   name = constant;
      | else
      |   const = str2num(constant);
      |   name = 'CONST';
      | end;
      mask Display: fprintf('%s = %.4f',name,const);
  CONSTANT9 : Subsystem  mask(Constant){constant=IDPPM_MAX__A}
      mask help: Constant Block. Will dispaly constant name and value on the icon of the block
      mask init:
      | if isletter(constant(1))
      |   const = evalin('base',constant);
      |   name = constant;
      | else
      |   const = str2num(constant);
      |   name = 'CONST';
      | end;
      mask Display: fprintf('%s = %.4f',name,const);
  Constant3 : Constant  Value=0.0
  Constant4 : Constant  Value=0.0
  Multiport Switch : MultiPortSwitch  Inputs=2
  Multiport Switch1 : MultiPortSwitch  Inputs=2
  Multiport Switch2 : MultiPortSwitch  Inputs=2
  Product7 : Product  Inputs=**  InputSameDT=on  RndMeth=Zero  SaturateOnIntegerOverflow=on  OutDataTypeStr=Inherit: Same as first input
  Terminator : Terminator
  Terminator1 : Terminator
  Unit Delay1 : UnitDelay  SampleTime=-1
  VAR_SATURATION1 : Subsystem  mask(VARIABLE SATURATION){}
      mask help: This block will clip the input between the MIN and MAX values specified as inputs to the block. In addition a LIMIT_FLAG will be set to 1 if the input is currently being clipped.
      mask Display:
      | plot( [0.2 0.3 0.5 0.6], [0.2 0.2 0.8 0.8])
      | text(0.2, 0.05, 'min')
      | text(0.5, 0.95, 'max')
  VAR_SATURATION2 : Subsystem  mask(VARIABLE SATURATION){}
      mask help: This block will clip the input between the MIN and MAX values specified as inputs to the block. In addition a LIMIT_FLAG will be set to 1 if the input is currently being clipped.
      mask Display:
      | plot( [0.2 0.3 0.5 0.6], [0.2 0.2 0.8 0.8])
      | text(0.2, 0.05, 'min')
      | text(0.5, 0.95, 'max')
  idle_ppm : Outport
  idnerr__A : Outport  Port=2
  wires:
  Multiport Switch1/1 -> Multiport Switch/2  "idnerr_db"
  [ml_init_sw] -> Multiport Switch2/1
  ml_init_sw/1 -> [ml_init_sw], Multiport Switch/1
  Multiport Switch/1 -> Unit Delay1/1, Product7/1, idnerr__A/1  "idnerr__A"
  VAR_SATURATION1/1(OUTPUT) -> VAR_SATURATION2/2(INPUT)  "id_prop_ppms__A"
  VAR_SATURATION2/1(OUTPUT) -> Multiport Switch2/2
  Multiport Switch2/1 -> idle_ppm/1  "idle_ppm"
  Constant4/1 -> Multiport Switch2/3
  VAR_SATURATION2/2(LIMIT_FLAG) -> Terminator1/1
  Constant3/1 -> VAR_SATURATION2/3(MIN)
  CONSTANT9/1(Out) -> VAR_SATURATION2/1(MAX)
  " 1"/1(Out1) -> Product7/2
  load/1 -> " 1"/1(In1)
  Product7/1 -> VAR_SATURATION1/2(INPUT)
  CONSTANT8/1(Out) -> VAR_SATURATION1/1(MAX)
  CONSTANT7/1(Out) -> VAR_SATURATION1/3(MIN)
  VAR_SATURATION1/2(LIMIT_FLAG) -> Terminator/1
  idnerr_fil/1 -> Multiport Switch1/2
  Unit Delay1/1 -> Multiport Switch1/3
  ml_idnerr_sw/1 -> Multiport Switch1/1
  ml_idnerr/1 -> Multiport Switch/3

== system mfordmodel_v1/iac_v04_001_001/normal_mode/iscflg_module/idle_drive_rpm_controller/idnerr_fil_calc ==
  ml_init_sw : Inport
  engine_speed : Inport  Port=2
  iac_dlt_time : Inport  Port=3
  do_idnerr_fil_calc : TriggerPort  TriggerType=function-call  VariantControl=(inherit)
  CONSTANT1 : Subsystem  mask(Constant){constant=ID_DSDRPM__A}
      mask help: Constant Block. Will dispaly constant name and value on the icon of the block
      mask init:
      | if isletter(constant(1))
      |   const = evalin('base',constant);
      |   name = constant;
      | else
      |   const = str2num(constant);
      |   name = 'CONST';
      | end;
      mask Display: fprintf('%s = %.4f',name,const);
  Multiport Switch1 : MultiPortSwitch  Inputs=2
  ROLAV_TC_DT_in1 : Subsystem  mask(Rolling Average - Time Constant){TAU=IDNERR_TC}
      mask prompts: TAU "Time Constant"
      mask help: Rolling Average - Time Constant. This filter block is the first order approximation using a time constant. Inputs include the time constant (entered through this dialogue), old_ave which is the previous average value, new_value which is the new filter to filter toward, and the delta_time which is elapsed time over which to perform the filter equation.
      mask init:
      | if isletter(TAU(1))
      |   tc = evalin('base',TAU);
      |   name = TAU;
      | else
      |   tc = str2num(TAU);
      |   name = 'TC';
      | end;
      mask Display: fprintf('%s = %.4f',name,tc);
  Sum8 : Sum  Inputs=+-  InputSameDT=on  SaturateOnIntegerOverflow=on  OutDataTypeStr=Inherit: Same as first input
  Unit Delay4 : UnitDelay  SampleTime=-1
  ml_idnerr : Outport
  idnerr_fil : Outport  Port=2
  wires:
  Unit Delay4/1 -> ROLAV_TC_DT_in1/2(old_ave)
  iac_dlt_time/1 -> ROLAV_TC_DT_in1/3(delta_time)
  CONSTANT1/1(Out) -> Sum8/1
  engine_speed/1 -> Sum8/2
  Sum8/1 -> ROLAV_TC_DT_in1/1(new_value), ml_idnerr/1, Multiport Switch1/3  "ml_idnerr"
  ROLAV_TC_DT_in1/1(new_ave) -> Multiport Switch1/2  "idnerr_fil"
  Multiport Switch1/1 -> idnerr_fil/1, Unit Delay4/1  "idnerr_fil"
  ml_init_sw/1 -> Multiport Switch1/1

== system mfordmodel_v1/iac_v04_001_001/normal_mode/iscflg_module/idle_rpm_controller/fn852a_calc ==
  ml_init_sw : Inport
  rpmerr : Inport  Port=2
  do_fn852a_calc : TriggerPort  TriggerType=function-call  VariantControl=(inherit)
  Constant2 : Constant  Value=0.0
  FN852A : Subsystem  mask(2-D, piece-wise, linear interpolation){CAL_FUNC=FN852A}
      mask prompts: CAL_FUNC "Calibration function name"
      mask help:
      | Performs piece-wise linear interpolation.
      |
      | Output is NOT extrapolated beyond the input range.  If the input value presented to the block lies outside the range specified in the block's parameter, then the value is treated as though it has the value of the nearest value in the range.
      mask init: same as mfordmodel_v1/iac_v04_001_001/activate_desired_rpm/rpm_calcs/lookup_2d
      mask Help:
      | Enter the name of the calibration function.
      | (e.g. EGM_VA_ECT_MULT)
      mask Display:
      | fprintf('%s',CAL_FUNC);
      | plot(calfunc.X,calfunc.Y,max_x*1.05,max_y*1.05,min_x,min_y);
  Multiport Switch2 : MultiPortSwitch  Inputs=2
  isc_a_prop_tmp : Outport
  wires:
  rpmerr/1 -> FN852A/1(In1)
  FN852A/1(Out1) -> Multiport Switch2/2
  Multiport Switch2/1 -> isc_a_prop_tmp/1  "isc_a_prop_tmp"
  ml_init_sw/1 -> Multiport Switch2/1
  Constant2/1 -> Multiport Switch2/3

== system mfordmodel_v1/iac_v04_001_001/normal_mode/iscflg_module/idle_rpm_controller/idle_ppm_calc ==
  ml_prop_sw : Inport
  ml_tcpro_sw : Inport  Port=2
  ml_der_sw : Inport  Port=3
  ml_init_sw : Inport  Port=4
  isc_a_prop_tmp : Inport  Port=5
  rpmerr : Inport  Port=6
  iac_dlt_time : Inport  Port=7
  do_idle_ppm_calc : TriggerPort  TriggerType=function-call  VariantControl=(inherit)
  Constant{1..4} (4 alike) : Constant  Value=0.0
  FN851A : Subsystem  mask(2-D, piece-wise, linear interpolation){CAL_FUNC=FN851A}
      mask prompts: CAL_FUNC "Calibration function name"
      mask help:
      | Performs piece-wise linear interpolation.
      |
      | Output is NOT extrapolated beyond the input range.  If the input value presented to the block lies outside the range specified in the block's parameter, then the value is treated as though it has the value of the nearest value in the range.
      mask init: same as mfordmodel_v1/iac_v04_001_001/activate_desired_rpm/rpm_calcs/lookup_2d
      mask Help:
      | Enter the name of the calibration function.
      | (e.g. EGM_VA_ECT_MULT)
      mask Display:
      | fprintf('%s',CAL_FUNC);
      | plot(calfunc.X,calfunc.Y,max_x*1.05,max_y*1.05,min_x,min_y);
  Multiport Switch{2..7} (6 alike) : MultiPortSwitch  Inputs=2
  PID_DELTA : Subsystem  mask(Constant){constant=PID_DELTA}
      mask help: Constant Block. Will dispaly constant name and value on the icon of the block
      mask init:
      | if isletter(constant(1))
      |   const = evalin('base',constant);
      |   name = constant;
      | else
      |   const = str2num(constant);
      |   name = 'CONST';
      | end;
      mask Display: fprintf('%s = %.4f',name,const);
  ROLAV_TC_in_DT_in : Subsystem  mask(Rolling Average - Time Constant){}
      mask help: Rolling Average - Time Constant. This filter block is the first order approximation using a time constant. Inputs include the time constant, old_ave which is the previous average value, new_value which is the new filter to filter toward, and the delta_time which is elapsed time over which to perform the filter equation.
      mask Display: fprintf('ROLAV_TC');
  ROLAV_TC_in_DT_in1 : Subsystem  mask(Rolling Average - Time Constant){}
      mask help: Rolling Average - Time Constant. This filter block is the first order approximation using a time constant. Inputs include the time constant, old_ave which is the previous average value, new_value which is the new filter to filter toward, and the delta_time which is elapsed time over which to perform the filter equation.
      mask Display: fprintf('ROLAV_TC');
  Sum1 : Sum  Inputs=+++  InputSameDT=on  SaturateOnIntegerOverflow=on  OutDataTypeStr=Inherit: Same as first input
  Sum2 : Sum  Inputs=+-  InputSameDT=on  SaturateOnIntegerOverflow=on  OutDataTypeStr=Inherit: Same as first input
  TCBPA_DER : Subsystem  mask(Constant){constant=TCBPA_DER}
      mask help: Constant Block. Will dispaly constant name and value on the icon of the block
      mask init:
      | if isletter(constant(1))
      |   const = evalin('base',constant);
      |   name = constant;
      | else
      |   const = str2num(constant);
      |   name = 'CONST';
      | end;
      mask Display: fprintf('%s = %.4f',name,const);
  TCPRO_GT : Subsystem  mask(Constant){constant=TCPRO_GT}
      mask help: Constant Block. Will dispaly constant name and value on the icon of the block
      mask init:
      | if isletter(constant(1))
      |   const = evalin('base',constant);
      |   name = constant;
      | else
      |   const = str2num(constant);
      |   name = 'CONST';
      | end;
      mask Display: fprintf('%s = %.4f',name,const);
  TCPRO_LT : Subsystem  mask(Constant){constant=TCPRO_LT}
      mask help: Constant Block. Will dispaly constant name and value on the icon of the block
      mask init:
      | if isletter(constant(1))
      |   const = evalin('base',constant);
      |   name = constant;
      | else
      |   const = str2num(constant);
      |   name = 'CONST';
      | end;
      mask Display: fprintf('%s = %.4f',name,const);
  Unit Delay : UnitDelay  SampleTime=-1
  Unit Delay1 : UnitDelay  SampleTime=-1
  idle_ppm : Outport
  isc_a_prop : Outport  Port=2
  wires:
  iac_dlt_time/1 -> [iac_dlt_time], ROLAV_TC_in_DT_in/4(delta_time)
  Multiport Switch2/1 -> isc_a_prop/1, Unit Delay/1, Sum1/1  "isc_a_prop"
  ml_init_sw/1 -> [ml_init_sw], Multiport Switch4/1
  Constant4/1 -> Multiport Switch7/3
  [ml_init_sw] -> Multiport Switch7/1
  Multiport Switch7/1 -> Unit Delay1/1  "rpmerr_da"
  ROLAV_TC_in_DT_in1/1(new_ave) -> Multiport Switch7/2
  ROLAV_TC_in_DT_in/1(new_ave) -> Multiport Switch2/2
  Constant3/1 -> Multiport Switch4/3
  FN851A/1(Out1) -> Multiport Switch4/2  "isc_a_der"
  Multiport Switch4/1 -> Sum1/3  "isc_a_der"
  PID_DELTA/1(Out) -> Sum1/2
  Sum2/1 -> FN851A/1(In1)
  Multiport Switch6/1 -> Sum2/1  "rpmerr_dao"
  rpmerr/1 -> Sum2/2, Multiport Switch6/2, ROLAV_TC_in_DT_in1/1(new_value)
  Unit Delay1/1 -> Multiport Switch6/3, ROLAV_TC_in_DT_in1/3(old_ave)
  ml_der_sw/1 -> Multiport Switch6/1, Multiport Switch5/1
  [iac_dlt_time] -> ROLAV_TC_in_DT_in1/4(delta_time)
  TCBPA_DER/1(Out) -> Multiport Switch5/3
  Constant2/1 -> Multiport Switch5/2
  Multiport Switch5/1 -> ROLAV_TC_in_DT_in1/2(Tau)
  Unit Delay/1 -> ROLAV_TC_in_DT_in/3(old_ave)
  TCPRO_LT/1(Out) -> Multiport Switch3/3
  ml_tcpro_sw/1 -> Multiport Switch3/1
  TCPRO_GT/1(Out) -> Multiport Switch3/2
  Multiport Switch3/1 -> ROLAV_TC_in_DT_in/2(Tau)
  Constant1/1 -> Multiport Switch2/3
  ml_prop_sw/1 -> Multiport Switch2/1
  Sum1/1 -> idle_ppm/1  "idle_ppm"
  isc_a_prop_tmp/1 -> ROLAV_TC_in_DT_in/1(new_value)

== system mfordmodel_v1/iac_v04_001_001/normal_mode/iscflg_module/idle_rpm_controller/ipsibr_calc ==
  ipsibr : Inport
  iscpsi : Inport  Port=2
  do_ipsibr_calc : TriggerPort  TriggerType=function-call  VariantControl=(inherit)
  Sum2 : Sum  InputSameDT=on  SaturateOnIntegerOverflow=on  OutDataTypeStr=Inherit: Same as first input
  ipsibr_fb : Outport
  wires:
  iscpsi/1 -> Sum2/2
  ipsibr/1 -> Sum2/1
  Sum2/1 -> ipsibr_fb/1  "ipsibr_fb"
